simulink model "Lab_5_Model_System"  (R2019b)
settings: Solver=ode45  StartTime=0.0  StopTime=240  MaxStep=0.01  RelTol=1e-6  AbsTol=1e-6
values from neighbouring files (symbols this model uses):
  alpha = 0    [procedure_5_1.m]    (also in procedure_5_2.m; procedure_5_3.m)
  delay = 6    [shared_variables.m]
  desired_offset = -5    [shared_variables.m]
  frequency = 100    [shared_variables.m]
  K = 0    [procedure_5_1.m]
  T = 0    [procedure_5_1.m]    (also in procedure_5_2.m; procedure_5_3.m)
settings Model: DataDictionary=Lab_5_Model_System_Data.sldd  Creator=rolle  LastModifiedBy=rollends
settings DataIOCC: SaveOutput=off  DSMLogging=off  SaveTime=off  ReturnWorkspaceOutputs=off

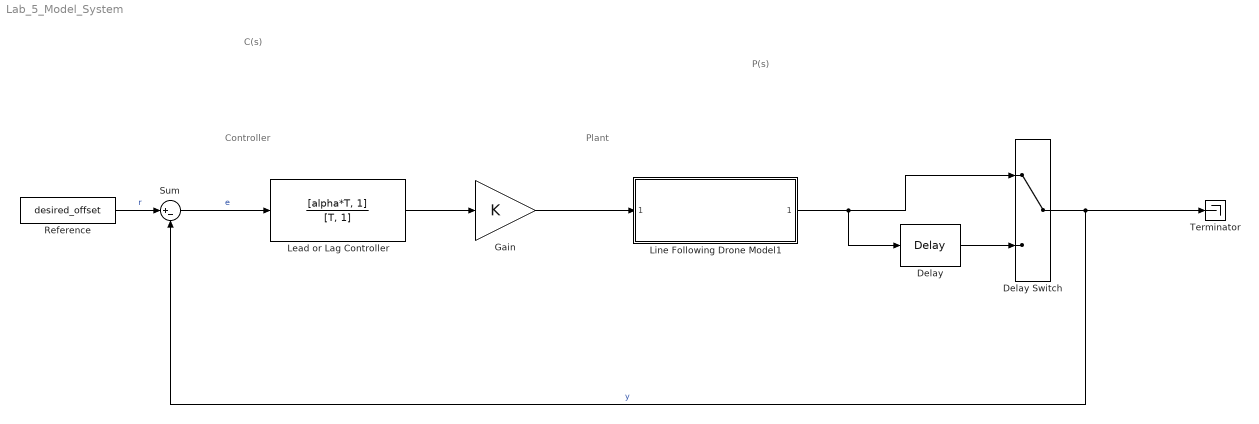
== system Lab_5_Model_System ==
  note: Plant
  note: Controller
  note: C(s)
  note: P(s)
  Delay : TransportDelay  DelayTime=delay/frequency  PadeOrder=4
  Delay Switch : ManualSwitch
  Gain : Gain  Gain=K
  Lead or Lag Controller : TransferFcn  Numerator=[alpha*T, 1]  Denominator=[T, 1]
  Line Following Drone Model1 : Subsystem  SCDEnableBlockLinearizationSpecification=on  ReferencedSubsystem=Line_Following_Drone_Model
  Reference : Constant  Value=desired_offset  OutDataTypeStr=Inherit: Inherit via back propagation
  Sum : Sum  Inputs=|+-
  Terminator : Terminator
  wires:
  Sum/1 -> Lead or Lag Controller/1  "e"
  Lead or Lag Controller/1 -> Gain/1
  Reference/1 -> Sum/1  "r"
  Delay Switch/1 -> Sum/2, Terminator/1  "y"
  Delay/1 -> Delay Switch/2
  Line Following Drone Model1/1 -> Delay/1, Delay Switch/1
  Gain/1 -> Line Following Drone Model1/1
